simulink model "angle_jiaozhen"  (R2021a)
settings: Solver=VariableStepAuto  StartTime=0.0  StopTime=10.0  RelTol=1e-3
settings Model: Creator=HanDong  LastModifiedBy=HanDong

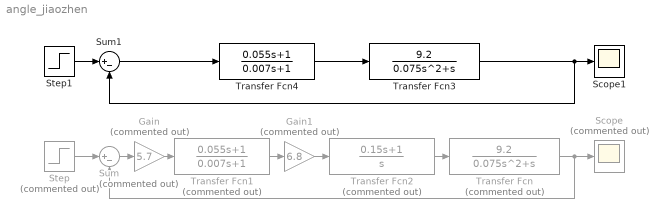
== system angle_jiaozhen ==
  Gain : Gain  Commented=on  Gain=5.7
  Gain1 : Gain  Commented=on  Gain=6.8
  Scope : Scope  Commented=on
  Scope1 : Scope
  Step : Step  Commented=on  SampleTime=0
  Step1 : Step  SampleTime=0
  Sum : Sum  Commented=on  Inputs=|+-
  Sum1 : Sum  Inputs=|+-
  Transfer Fcn : TransferFcn  Commented=on  Numerator=[9.2]  Denominator=[0.075 1 0]
  Transfer Fcn1 : TransferFcn  Commented=on  Numerator=[0.055 1]  Denominator=[0.007 1]
  Transfer Fcn2 : TransferFcn  Commented=on  Numerator=[0.15 1]  Denominator=[1 0]
  Transfer Fcn3 : TransferFcn  Numerator=[9.2]  Denominator=[0.075 1 0]
  Transfer Fcn4 : TransferFcn  Numerator=[0.055 1]  Denominator=[0.007 1]
  wires:
  Step/1 -> Sum/1
  Sum/1 -> Gain/1
  Transfer Fcn2/1 -> Transfer Fcn/1
  Transfer Fcn/1 -> Sum/2, Scope/1
  Gain/1 -> Transfer Fcn1/1
  Transfer Fcn1/1 -> Gain1/1
  Gain1/1 -> Transfer Fcn2/1
  Transfer Fcn3/1 -> Sum1/2, Scope1/1
  Transfer Fcn4/1 -> Transfer Fcn3/1
  Sum1/1 -> Transfer Fcn4/1
  Step1/1 -> Sum1/1
